simulink library "structure_lib"  (R2018b)
settings: Solver=VariableStepAuto  StartTime=0.0  StopTime=10.0  RelTol=1e-3
values from neighbouring files (symbols this model uses):
  structure = structureSetNodeCg( structure, 1:num_nodes, cg_node )    [structureScale.m]
  structure_red = structure    [structurePlotEigenmode.m]
undefined symbols (not defined in the file or in its folder): config, structureGetNodeInertiaRef, structureGetNodeMass
libraries: axes_transformation_lib x1
settings Model: Creator=Ybeyer  LastModifiedBy=Yannic
settings SFSimCC: SimUseLocalCustomCode=off
settings RTWCC: RTWUseLocalCustomCode=off
settings CodeAppCC: StateflowObjectComments=on

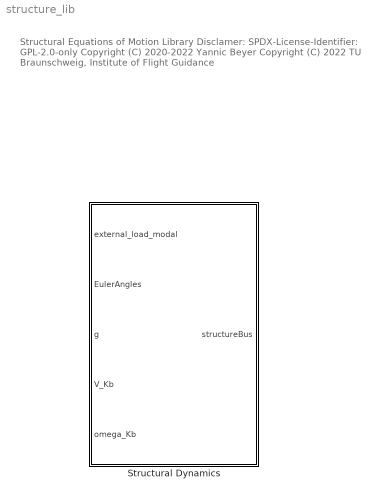
== system structure_lib ==
  note: Structural Equations of Motion Library
      |
      | Disclamer:
      | SPDX-License-Identifier: GPL-2.0-only
      |
      | Copyright (C) 2020-2022 Yannic Beyer
      | Copyright (C) 2022 TU Braunschweig, Institute of Flight Guidance
  Structural Dynamics : Subsystem  mask{structure_vel_0=zeros( size( structure_red.K, 1) - 6, 1 ), structure_pos_0=zeros( size( structure_red.K, 1) - 6, 1 ), r_nodes=structure.xyz-repmat(config.xyz_ref_c,1,size(structure.xyz,2)), m_nodes=structureGetNodeMass(structure,1:size(structure.xyz,2)), I_nodes=reshape(permute(structureGetNodeInertiaRef(structure,1:size(structure.xyz,2),config.xyz_ref_c),[2,1,3]),3,[])', K=structure_red.K, M=structure_red.M, T_structure=structure_red.modal.T, T_ref=config.T_ref_s}
      mask prompts: structure_vel_0 "initial structure velocity"; structure_pos_0 "initial structure (Delta) position"; r_nodes "concentrated position vectors of nodes in reference axis (3xn)"; m_nodes "mass vector of all nodes"; I_nodes "concentrated inertia matrices of all notes w.r.t. reference axis (3*N x 3)"; K "stiffness matrix"; M "mass matrix"; T_structure "transformation matrix from nodes to state vector (e.g. generalized coordinates), see structureGetReduced"; T_ref "transformation matrix from structure state to reference point, see structureGetRefPointTrafo"
      mask DialogControl DescGroupVar Prompt: Structural Dynamics
      mask DialogControl DescTextVar Prompt: Computes acceleration of reference point for rigid body equations of motion
      mask DialogControl Control2 Prompt: as well as the structure state which can be fed back to the aerodynamics model.
      mask DialogControl Control3 Prompt: First six states of structural dynamics model are considered to be the rigid body states.

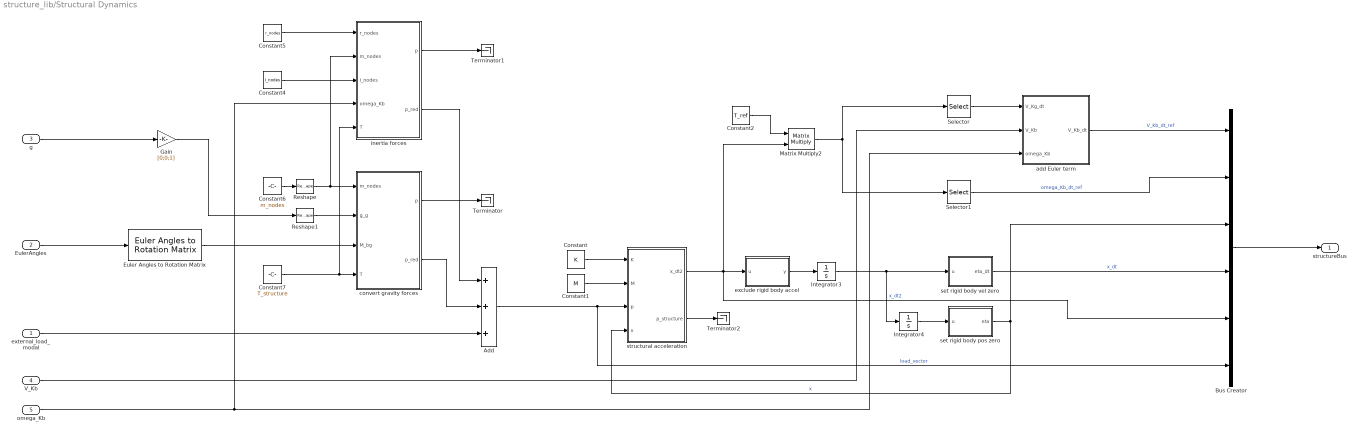
== system structure_lib/Structural Dynamics ==
  external_load_modal : Inport
  EulerAngles : Inport  Port=2
  g : Inport  Port=3
  V_Kb : Inport  Port=4
  omega_Kb : Inport  Port=5
  Add : Sum  Inputs=+++
  Bus Creator : BusCreator  Inputs=6
  Constant : Constant  Value=K
  Constant1 : Constant  Value=M
  Constant2 : Constant  Value=T_ref
  Constant4 : Constant  Value=I_nodes  OutDataTypeStr=Inherit: Inherit via back propagation
  Constant5 : Constant  Value=r_nodes
  Constant6 : Constant  Value=m_nodes  OutDataTypeStr=Inherit: Inherit via back propagation
  Constant7 : Constant  Value=T_structure
  Euler Angles to Rotation Matrix : axes_transformation_lib/Euler Angles to Rotation Matrix  SystemSampleTime=-1
      settings: SourceProductName=LADAC
  Gain : Gain  Gain=[0;0;1]
  Integrator3 : Integrator  InitialCondition=structure_vel_0
  Integrator4 : Integrator  InitialCondition=structure_pos_0
  Matrix Multiply2 : Product  Multiplication=Matrix(*)
  Reshape : Reshape  OutputDimensionality=Row vector (2-D)
  Reshape1 : Reshape  OutputDimensionality=Column vector (2-D)
  Selector : Selector  InputPortWidth=6  IndexOptions=Index vector (dialog)  Indices=[1:3]  OutputSizes=1
  Selector1 : Selector  InputPortWidth=6  IndexOptions=Index vector (dialog)  Indices=[4:6]  OutputSizes=1
  Terminator : Terminator
  Terminator1 : Terminator
  Terminator2 : Terminator
  add Euler term : MATLAB Function  TreatAsAtomicUnit=on
  convert gravity forces : MATLAB Function  TreatAsAtomicUnit=on
  exclude rigid body accel : MATLAB Function  TreatAsAtomicUnit=on
  inertia forces : MATLAB Function  TreatAsAtomicUnit=on
  set rigid body pos zero : MATLAB Function  TreatAsAtomicUnit=on
  set rigid body vel zero : MATLAB Function  TreatAsAtomicUnit=on
  structural acceleration : MATLAB Function  TreatAsAtomicUnit=on
  structureBus : Outport
  wires:
  Constant/1 -> structural acceleration/1(K)
  Add/1 -> Bus Creator/6, structural acceleration/3(p)  "load_vector"
  Constant1/1 -> structural acceleration/2(M)
  EulerAngles/1 -> Euler Angles to Rotation Matrix/1
  Euler Angles to Rotation Matrix/1 -> convert gravity forces/3(M_bg)
  Gain/1 -> Reshape1/1
  Constant6/1 -> Reshape/1
  convert gravity forces/2(p_red) -> Add/2
  Constant7/1 -> convert gravity forces/4(T), inertia forces/5(T)
  structural acceleration/1(x_dt2) -> Bus Creator/5, exclude rigid body accel/1(u), Matrix Multiply2/2  "x_dt2"
  Constant2/1 -> Matrix Multiply2/1
  Matrix Multiply2/1 -> Selector/1, Selector1/1
  convert gravity forces/1(p) -> Terminator/1
  exclude rigid body accel/1(y) -> Integrator3/1
  Integrator3/1 -> set rigid body vel zero/1(u), Integrator4/1
  Integrator4/1 -> set rigid body pos zero/1(u)
  set rigid body vel zero/1(eta_dt) -> Bus Creator/4  "x_dt"
  set rigid body pos zero/1(eta) -> Bus Creator/3, structural acceleration/4(x)  "x"
  Selector/1 -> add Euler term/1(V_Kg_dt)
  external_load_modal/1 -> Add/3
  g/1 -> Gain/1
  Reshape1/1 -> convert gravity forces/2(g_g)
  add Euler term/1(V_Kb_dt) -> Bus Creator/1  "V_Kb_dt_ref"
  Selector1/1 -> Bus Creator/2  "omega_Kb_dt_ref"
  V_Kb/1 -> add Euler term/2(V_Kb)
  omega_Kb/1 -> add Euler term/3(omega_Kb), inertia forces/4(omega_Kb)
  Constant4/1 -> inertia forces/3(I_nodes)
  Constant5/1 -> inertia forces/1(r_nodes)
  inertia forces/1(p) -> Terminator1/1
  Reshape/1 -> convert gravity forces/1(m_nodes), inertia forces/2(m_nodes)
  inertia forces/2(p_red) -> Add/1
  Bus Creator/1 -> structureBus/1
  structural acceleration/2(p_structure) -> Terminator2/1

== matlab function structure_lib/Structural Dynamics/inertia forces ==
  data: r_nodes input; p output; m_nodes input; I_nodes input; p_red output; omega_Kb input; T input
function [p,p_red] = fcn(r_nodes, m_nodes, I_nodes, omega_Kb, T)

% Which forces are required?
% 
% Nomenclature:
%   m               mass of object
%   r               position vector of object in inertial system S
%   r'              relative position vector of object in local system S'
%   v=r_dt          velocity of object in S
%   v'              relative velocity of object in S'
%   a=v_dt          acceleration of object in S
%   a'              relative acceleration of object in S'
%   r_B             position of origin of S' in S
%   v_B = r_B_dt    velocity of origin of S' in S
%   a_B = v_B_dt    acceleration of origin of S' in S
%   w               angular velocity vector of S' in S
%   w_dt            angular acceleration of S' in S
%   x               cross product
%   
% Motion of local system:
%   r = r_b + r'
%   v = r_dt = v_B + wxr' + v'
%   a = v_dt = a_B + wx(wxr') + w_dtxr' + 2*wxv' + a'
% 
%   m*a' = F - m*a_B - m*wx(wxr') - m*w_dtxr' - 2*m*wxv'
% 
%   -m*wx(wxr')     centrifugal force
%   -m*w_dtxr'      Euler force
%   -2*m*wxv'       Coriolis force
% 
% Assumptions:
%   1)  a' and w_dt(w=0) are obtained by by solving the free structural model:
%       b' = inv(M) * ( p - K*x )
%           where
%           p is the load vector,
%           M is the mass matrix,
%           K is the stiffness matrix,
%           x is the deformation vector,
%           b'(6*(N-1)+1,6*(N-1)+2,6*(N-1)+3) = a'(N,N+1,N+2),
%           b'(6*(N-1)+4,6*(N-1)+5,6*(N-1)+6) = w_dt(N+3,N+4,N+5),
%           N is the number of the node.
%   2)  Euler force for the part w_dt(w=0) must not be considered because
%       it is considered indirectly by 1) (?).
%       For the Euler force, w_dt = -inv(I)*(wxI*w), where I is the inertia
%       of the object w.r.t. S'.
%   3)  Coriolis force can be neglected
%   

n_nodes = size(m_nodes,2);

% Euler force due to rotation of the reference frame w.r.t. inertial
% frame
I = [ sum(I_nodes(1:3:end,:),1); sum(I_nodes(2:3:end,:),1); sum(I_nodes(3:3:end,:),1) ];
I_inv = inv(I);
p_Euler_b = [ ...
    -cross( matrixMultiplyNd( I_inv, ...
    cross( omega_Kb * m_nodes , reshape( I_nodes * omega_Kb, 3, [] ), 1 ) ), ...
    r_nodes, 1 ); ...
    zeros(3,size(m_nodes,2)) ...
    ];

% centrifugal force due to rotation of reference frame w.r.t. inertial
% frame
p_centrifugal_b = [ ...
    -cross( omega_Kb*m_nodes, cross( repmat(omega_Kb,1,n_nodes), r_nodes, 1 ) ); ...
    zeros(3,n_nodes) ...
    ];

p_6xn = p_Euler_b + p_centrifugal_b;

p = reshape( p_6xn, [], 1 );

p_red = T' * p;

end

== matlab function structure_lib/Structural Dynamics/add Euler term ==
  data: V_Kg_dt input; V_Kb_dt output; V_Kb input; omega_Kb input
function V_Kb_dt  = fcn( V_Kg_dt, V_Kb, omega_Kb )

% add Euler term
V_Kb_dt = V_Kg_dt - cross( omega_Kb, V_Kb );

end

== matlab function structure_lib/Structural Dynamics/convert gravity forces ==
  data: p output; m_nodes input; p_red output; g_g input; M_bg input; T input
function [p,p_red] = fcn( m_nodes, g_g, M_bg, T )

g_b = M_bg * g_g;

% force of gravity
p_gravity_b = [ ...
    g_b * m_nodes; ...
    zeros(3,size(m_nodes,2)) ...
    ];

p = reshape( p_gravity_b, [], 1 );

p_red = T' * p;

end

== matlab function structure_lib/Structural Dynamics/structural acceleration ==
  data: K input; x_dt2 output; M input; p input; x input; p_structure output
function [x_dt2,p_structure] = fcn(K, M, p, x) %#codegen
p_structure = K*x;
x_dt2 = M \ (p-p_structure);
end

== matlab function structure_lib/Structural Dynamics/exclude rigid body accel ==
  data: u input; y output
function y = fcn(u) %#codegen
y = u(7:end);
end

== matlab function structure_lib/Structural Dynamics/set rigid body vel zero ==
  data: u input; eta_dt output
function eta_dt = fcn(u) %#codegen
eta_dt = [zeros(6,1);u];
end

== matlab function structure_lib/Structural Dynamics/set rigid body pos zero ==
  data: u input; eta output
function eta = fcn(u) %#codegen
eta = [zeros(6,1);u];
end
